simulink model "DC_MOTORControl2"  (R2021a)
settings: Solver=VariableStepAuto  StartTime=0.0  StopTime=1580  RelTol=1e-3
values from neighbouring files (symbols this model uses):
  B = 0.029    [MAIN.m]
  conv = 2*pi*2000    (= 12566.3706144)    [MAIN.m]
  J = 0.1    [MAIN.m]
  K = Ke    (= 0.6)    [MAIN.m]
  Ke = 0.6    [MAIN.m]
  Kt = 0.6    [MAIN.m]
  La = 1e-3    (= 0.001)    [MAIN.m]
  Ra = 1    [MAIN.m]
libraries: pid_lib x6, simulink x1
settings Model: Creator=Ferna  LastModifiedBy=Ferna

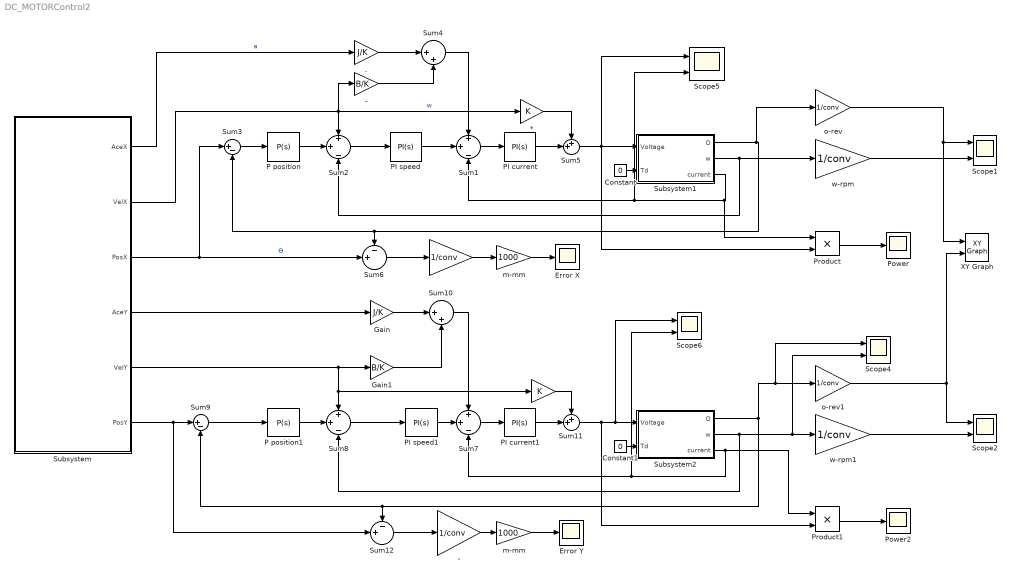
== system DC_MOTORControl2 ==
  " " : Gain  Gain=K
  "  " : Gain  Gain=1/conv
  ' : Gain  Gain=1/conv
  * : Gain  Gain=K
  - : Gain  Gain=B/K
  . : Gain  Gain=J/K
  Constant : Constant  Value=0
  Constant1 : Constant  Value=0
  Error X : Scope
  Error Y : Scope
  Gain : Gain  Gain=J/K
  Gain1 : Gain  Gain=B/K
  P position : pid_lib/PID Controller  Controller=P  Form=Parallel  TimeDomain=Continuous-time  UseExternalTs=off  SampleTime=-1  IntegratorMethod=Forward Euler  FilterMethod=Forward Euler  ControllerParametersSource=internal  P=1.1  I=B*5  D=0  UseFilter=on  N=100  TunerSelectOption=Transfer Function Based (PID Tuner App)  InitialConditionSource=internal  InitialConditionForIntegrator=0  InitialConditionForFilter=0  DifferentiatorICPrevScaledInput=0  ExternalReset=none  TrackingMode=off  Kt=1  LimitOutput=off  SatLimitsSource=internal  UpperSaturationLimit=inf  LowerSaturationLimit=-inf  LinearizeAsGain=on  AntiWindupMode=none  Kb=1  POutMin=[]  POutMax=[]  IOutMin=[]  IOutMax=[]  DOutMin=[]  DOutMax=[]  NOutMin=[]  NOutMax=[]  SumOutMin=[]  SumOutMax=[]  SaturationOutMin=[]  SaturationOutMax=[]  PParamMin=[]  PParamMax=[]  IParamMin=[]  IParamMax=[]  DParamMin=[]  DParamMax=[]  NParamMin=[]  NParamMax=[]  KbParamMin=[]  KbParamMax=[]  KtParamMin=[]  KtParamMax=[]  KbOutMin=[]  KbOutMax=[]  KtOutMin=[]  KtOutMax=[]  IntegratorOutMin=[]  IntegratorOutMax=[]  FilterOutMin=[]  FilterOutMax=[]  SumI1OutMin=[]  SumI1OutMax=[]  SumI2OutMin=[]  SumI2OutMax=[]  SumI3OutMin=[]  SumI3OutMax=[]  SumI4OutMin=[]  SumI4OutMax=[]  SumDOutMin=[]  SumDOutMax=[]  DifferentiatorOutMin=[]  DifferentiatorOutMax=[]  FilterDiffOutCoefMin=[]  FilterDiffOutCoefMax=[]  ReciprocalOutMin=[]  ReciprocalOutMax=[]  SumDenOutMin=[]  SumDenOutMax=[]  SumNumOutMin=[]  SumNumOutMax=[]  DivideOutMin=[]  DivideOutMax=[]  UdiffTsProdOutMin=[]  UdiffTsProdOutMax=[]  NTsProdOutMin=[]  NTsProdOutMax=[]  UintegralTsProdOutMin=[]  UintegralTsProdOutMax=[]  UngainTsProdOutMin=[]  UngainTsProdOutMax=[]  IntegratorContinuousStateAttributes=''  IntegratorStateMustResolveToSignalObject=off  IntegratorRTWStateStorageClass=Auto  FilterContinuousStateAttributes=''  FilterStateMustResolveToSignalObject=off  FilterRTWStateStorageClass=Auto  ParallelPVariant=InternalParameters  IdealPVariant=Disabled  IVariant=Disabled  DVariant=Disabled  IntegratorVariant=Disabled  SatVariant=Disabled  AWVariant=Disabled  PCopyVariant=Disabled  TRVariant=Disabled  FdbkBlocksVariant=Forward  IdealPFdbkVariant=Disabled  SatFdbkVariant=Disabled  DerivativeFilterVariant=Disabled  NVariant=Disabled  NCopyVariant=Disabled_SignalSpec  FilterICVariant=Disabled  IntegratorICVariant=Disabled  ExternalResetVariant=Disabled  TRSumVariant=Passthrough  SumFdbkVariant=Disabled  SumVariant=Passthrough_P  TsampFilterVariant=InternalTs  TsampNgainVariant=Passthrough  TsampIntegralVariant=Disabled_SignalSpec  ExternalSaturationOutDataTypeStr=Inherit: Same as second input
  P position1 : pid_lib/PID Controller  Controller=P  Form=Parallel  TimeDomain=Continuous-time  UseExternalTs=off  SampleTime=-1  IntegratorMethod=Forward Euler  FilterMethod=Forward Euler  ControllerParametersSource=internal  P=1.1  I=B*5  D=0  UseFilter=on  N=100  TunerSelectOption=Transfer Function Based (PID Tuner App)  InitialConditionSource=internal  InitialConditionForIntegrator=0  InitialConditionForFilter=0  DifferentiatorICPrevScaledInput=0  ExternalReset=none  TrackingMode=off  Kt=1  LimitOutput=off  SatLimitsSource=internal  UpperSaturationLimit=inf  LowerSaturationLimit=-inf  LinearizeAsGain=on  AntiWindupMode=none  Kb=1  POutMin=[]  POutMax=[]  IOutMin=[]  IOutMax=[]  DOutMin=[]  DOutMax=[]  NOutMin=[]  NOutMax=[]  SumOutMin=[]  SumOutMax=[]  SaturationOutMin=[]  SaturationOutMax=[]  PParamMin=[]  PParamMax=[]  IParamMin=[]  IParamMax=[]  DParamMin=[]  DParamMax=[]  NParamMin=[]  NParamMax=[]  KbParamMin=[]  KbParamMax=[]  KtParamMin=[]  KtParamMax=[]  KbOutMin=[]  KbOutMax=[]  KtOutMin=[]  KtOutMax=[]  IntegratorOutMin=[]  IntegratorOutMax=[]  FilterOutMin=[]  FilterOutMax=[]  SumI1OutMin=[]  SumI1OutMax=[]  SumI2OutMin=[]  SumI2OutMax=[]  SumI3OutMin=[]  SumI3OutMax=[]  SumI4OutMin=[]  SumI4OutMax=[]  SumDOutMin=[]  SumDOutMax=[]  DifferentiatorOutMin=[]  DifferentiatorOutMax=[]  FilterDiffOutCoefMin=[]  FilterDiffOutCoefMax=[]  ReciprocalOutMin=[]  ReciprocalOutMax=[]  SumDenOutMin=[]  SumDenOutMax=[]  SumNumOutMin=[]  SumNumOutMax=[]  DivideOutMin=[]  DivideOutMax=[]  UdiffTsProdOutMin=[]  UdiffTsProdOutMax=[]  NTsProdOutMin=[]  NTsProdOutMax=[]  UintegralTsProdOutMin=[]  UintegralTsProdOutMax=[]  UngainTsProdOutMin=[]  UngainTsProdOutMax=[]  IntegratorContinuousStateAttributes=''  IntegratorStateMustResolveToSignalObject=off  IntegratorRTWStateStorageClass=Auto  FilterContinuousStateAttributes=''  FilterStateMustResolveToSignalObject=off  FilterRTWStateStorageClass=Auto  ParallelPVariant=InternalParameters  IdealPVariant=Disabled  IVariant=Disabled  DVariant=Disabled  IntegratorVariant=Disabled  SatVariant=Disabled  AWVariant=Disabled  PCopyVariant=Disabled  TRVariant=Disabled  FdbkBlocksVariant=Forward  IdealPFdbkVariant=Disabled  SatFdbkVariant=Disabled  DerivativeFilterVariant=Disabled  NVariant=Disabled  NCopyVariant=Disabled_SignalSpec  FilterICVariant=Disabled  IntegratorICVariant=Disabled  ExternalResetVariant=Disabled  TRSumVariant=Passthrough  SumFdbkVariant=Disabled  SumVariant=Passthrough_P  TsampFilterVariant=InternalTs  TsampNgainVariant=Passthrough  TsampIntegralVariant=Disabled_SignalSpec  ExternalSaturationOutDataTypeStr=Inherit: Same as second input
  PI current : pid_lib/PID Controller  Controller=PI  Form=Parallel  TimeDomain=Continuous-time  UseExternalTs=off  SampleTime=-1  IntegratorMethod=Forward Euler  FilterMethod=Forward Euler  ControllerParametersSource=internal  P=La*1000  I=Ra*1000  D=0  UseFilter=on  N=100  TunerSelectOption=Transfer Function Based (PID Tuner App)  InitialConditionSource=internal  InitialConditionForIntegrator=0  InitialConditionForFilter=0  DifferentiatorICPrevScaledInput=0  ExternalReset=none  TrackingMode=off  Kt=1  LimitOutput=off  SatLimitsSource=internal  UpperSaturationLimit=inf  LowerSaturationLimit=-inf  LinearizeAsGain=on  AntiWindupMode=none  Kb=1  POutMin=[]  POutMax=[]  IOutMin=[]  IOutMax=[]  DOutMin=[]  DOutMax=[]  NOutMin=[]  NOutMax=[]  SumOutMin=[]  SumOutMax=[]  SaturationOutMin=[]  SaturationOutMax=[]  PParamMin=[]  PParamMax=[]  IParamMin=[]  IParamMax=[]  DParamMin=[]  DParamMax=[]  NParamMin=[]  NParamMax=[]  KbParamMin=[]  KbParamMax=[]  KtParamMin=[]  KtParamMax=[]  KbOutMin=[]  KbOutMax=[]  KtOutMin=[]  KtOutMax=[]  IntegratorOutMin=[]  IntegratorOutMax=[]  FilterOutMin=[]  FilterOutMax=[]  SumI1OutMin=[]  SumI1OutMax=[]  SumI2OutMin=[]  SumI2OutMax=[]  SumI3OutMin=[]  SumI3OutMax=[]  SumI4OutMin=[]  SumI4OutMax=[]  SumDOutMin=[]  SumDOutMax=[]  DifferentiatorOutMin=[]  DifferentiatorOutMax=[]  FilterDiffOutCoefMin=[]  FilterDiffOutCoefMax=[]  ReciprocalOutMin=[]  ReciprocalOutMax=[]  SumDenOutMin=[]  SumDenOutMax=[]  SumNumOutMin=[]  SumNumOutMax=[]  DivideOutMin=[]  DivideOutMax=[]  UdiffTsProdOutMin=[]  UdiffTsProdOutMax=[]  NTsProdOutMin=[]  NTsProdOutMax=[]  UintegralTsProdOutMin=[]  UintegralTsProdOutMax=[]  UngainTsProdOutMin=[]  UngainTsProdOutMax=[]  IntegratorContinuousStateAttributes=''  IntegratorStateMustResolveToSignalObject=off  IntegratorRTWStateStorageClass=Auto  FilterContinuousStateAttributes=''  FilterStateMustResolveToSignalObject=off  FilterRTWStateStorageClass=Auto  ParallelPVariant=InternalParameters  IdealPVariant=Disabled  IVariant=InternalParameters  DVariant=Disabled  IntegratorVariant=Continuous  SatVariant=Disabled  AWVariant=Passthrough  PCopyVariant=Disabled  TRVariant=Disabled  FdbkBlocksVariant=Forward  IdealPFdbkVariant=Disabled  SatFdbkVariant=Disabled  DerivativeFilterVariant=Disabled  NVariant=Disabled  NCopyVariant=Disabled_SignalSpec  FilterICVariant=Disabled  IntegratorICVariant=InternalICs  ExternalResetVariant=Disabled  TRSumVariant=Passthrough  SumFdbkVariant=Disabled  SumVariant=Sum_PI  TsampFilterVariant=InternalTs  TsampNgainVariant=Passthrough  TsampIntegralVariant=Passthrough  ExternalSaturationOutDataTypeStr=Inherit: Same as second input
  PI current1 : pid_lib/PID Controller  Controller=PI  Form=Parallel  TimeDomain=Continuous-time  UseExternalTs=off  SampleTime=-1  IntegratorMethod=Forward Euler  FilterMethod=Forward Euler  ControllerParametersSource=internal  P=La*1000  I=Ra*1000  D=0  UseFilter=on  N=100  TunerSelectOption=Transfer Function Based (PID Tuner App)  InitialConditionSource=internal  InitialConditionForIntegrator=0  InitialConditionForFilter=0  DifferentiatorICPrevScaledInput=0  ExternalReset=none  TrackingMode=off  Kt=1  LimitOutput=off  SatLimitsSource=internal  UpperSaturationLimit=inf  LowerSaturationLimit=-inf  LinearizeAsGain=on  AntiWindupMode=none  Kb=1  POutMin=[]  POutMax=[]  IOutMin=[]  IOutMax=[]  DOutMin=[]  DOutMax=[]  NOutMin=[]  NOutMax=[]  SumOutMin=[]  SumOutMax=[]  SaturationOutMin=[]  SaturationOutMax=[]  PParamMin=[]  PParamMax=[]  IParamMin=[]  IParamMax=[]  DParamMin=[]  DParamMax=[]  NParamMin=[]  NParamMax=[]  KbParamMin=[]  KbParamMax=[]  KtParamMin=[]  KtParamMax=[]  KbOutMin=[]  KbOutMax=[]  KtOutMin=[]  KtOutMax=[]  IntegratorOutMin=[]  IntegratorOutMax=[]  FilterOutMin=[]  FilterOutMax=[]  SumI1OutMin=[]  SumI1OutMax=[]  SumI2OutMin=[]  SumI2OutMax=[]  SumI3OutMin=[]  SumI3OutMax=[]  SumI4OutMin=[]  SumI4OutMax=[]  SumDOutMin=[]  SumDOutMax=[]  DifferentiatorOutMin=[]  DifferentiatorOutMax=[]  FilterDiffOutCoefMin=[]  FilterDiffOutCoefMax=[]  ReciprocalOutMin=[]  ReciprocalOutMax=[]  SumDenOutMin=[]  SumDenOutMax=[]  SumNumOutMin=[]  SumNumOutMax=[]  DivideOutMin=[]  DivideOutMax=[]  UdiffTsProdOutMin=[]  UdiffTsProdOutMax=[]  NTsProdOutMin=[]  NTsProdOutMax=[]  UintegralTsProdOutMin=[]  UintegralTsProdOutMax=[]  UngainTsProdOutMin=[]  UngainTsProdOutMax=[]  IntegratorContinuousStateAttributes=''  IntegratorStateMustResolveToSignalObject=off  IntegratorRTWStateStorageClass=Auto  FilterContinuousStateAttributes=''  FilterStateMustResolveToSignalObject=off  FilterRTWStateStorageClass=Auto  ParallelPVariant=InternalParameters  IdealPVariant=Disabled  IVariant=InternalParameters  DVariant=Disabled  IntegratorVariant=Continuous  SatVariant=Disabled  AWVariant=Passthrough  PCopyVariant=Disabled  TRVariant=Disabled  FdbkBlocksVariant=Forward  IdealPFdbkVariant=Disabled  SatFdbkVariant=Disabled  DerivativeFilterVariant=Disabled  NVariant=Disabled  NCopyVariant=Disabled_SignalSpec  FilterICVariant=Disabled  IntegratorICVariant=InternalICs  ExternalResetVariant=Disabled  TRSumVariant=Passthrough  SumFdbkVariant=Disabled  SumVariant=Sum_PI  TsampFilterVariant=InternalTs  TsampNgainVariant=Passthrough  TsampIntegralVariant=Passthrough  ExternalSaturationOutDataTypeStr=Inherit: Same as second input
  PI speed : pid_lib/PID Controller  Controller=PI  Form=Parallel  TimeDomain=Continuous-time  UseExternalTs=off  SampleTime=-1  IntegratorMethod=Forward Euler  FilterMethod=Forward Euler  ControllerParametersSource=internal  P=J*10  I=B*10  D=0  UseFilter=on  N=100  TunerSelectOption=Transfer Function Based (PID Tuner App)  InitialConditionSource=internal  InitialConditionForIntegrator=0  InitialConditionForFilter=0  DifferentiatorICPrevScaledInput=0  ExternalReset=none  TrackingMode=off  Kt=1  LimitOutput=off  SatLimitsSource=internal  UpperSaturationLimit=inf  LowerSaturationLimit=-inf  LinearizeAsGain=on  AntiWindupMode=none  Kb=1  POutMin=[]  POutMax=[]  IOutMin=[]  IOutMax=[]  DOutMin=[]  DOutMax=[]  NOutMin=[]  NOutMax=[]  SumOutMin=[]  SumOutMax=[]  SaturationOutMin=[]  SaturationOutMax=[]  PParamMin=[]  PParamMax=[]  IParamMin=[]  IParamMax=[]  DParamMin=[]  DParamMax=[]  NParamMin=[]  NParamMax=[]  KbParamMin=[]  KbParamMax=[]  KtParamMin=[]  KtParamMax=[]  KbOutMin=[]  KbOutMax=[]  KtOutMin=[]  KtOutMax=[]  IntegratorOutMin=[]  IntegratorOutMax=[]  FilterOutMin=[]  FilterOutMax=[]  SumI1OutMin=[]  SumI1OutMax=[]  SumI2OutMin=[]  SumI2OutMax=[]  SumI3OutMin=[]  SumI3OutMax=[]  SumI4OutMin=[]  SumI4OutMax=[]  SumDOutMin=[]  SumDOutMax=[]  DifferentiatorOutMin=[]  DifferentiatorOutMax=[]  FilterDiffOutCoefMin=[]  FilterDiffOutCoefMax=[]  ReciprocalOutMin=[]  ReciprocalOutMax=[]  SumDenOutMin=[]  SumDenOutMax=[]  SumNumOutMin=[]  SumNumOutMax=[]  DivideOutMin=[]  DivideOutMax=[]  UdiffTsProdOutMin=[]  UdiffTsProdOutMax=[]  NTsProdOutMin=[]  NTsProdOutMax=[]  UintegralTsProdOutMin=[]  UintegralTsProdOutMax=[]  UngainTsProdOutMin=[]  UngainTsProdOutMax=[]  IntegratorContinuousStateAttributes=''  IntegratorStateMustResolveToSignalObject=off  IntegratorRTWStateStorageClass=Auto  FilterContinuousStateAttributes=''  FilterStateMustResolveToSignalObject=off  FilterRTWStateStorageClass=Auto  ParallelPVariant=InternalParameters  IdealPVariant=Disabled  IVariant=InternalParameters  DVariant=Disabled  IntegratorVariant=Continuous  SatVariant=Disabled  AWVariant=Passthrough  PCopyVariant=Disabled  TRVariant=Disabled  FdbkBlocksVariant=Forward  IdealPFdbkVariant=Disabled  SatFdbkVariant=Disabled  DerivativeFilterVariant=Disabled  NVariant=Disabled  NCopyVariant=Disabled_SignalSpec  FilterICVariant=Disabled  IntegratorICVariant=InternalICs  ExternalResetVariant=Disabled  TRSumVariant=Passthrough  SumFdbkVariant=Disabled  SumVariant=Sum_PI  TsampFilterVariant=InternalTs  TsampNgainVariant=Passthrough  TsampIntegralVariant=Passthrough  ExternalSaturationOutDataTypeStr=Inherit: Same as second input
  PI speed1 : pid_lib/PID Controller  Controller=PI  Form=Parallel  TimeDomain=Continuous-time  UseExternalTs=off  SampleTime=-1  IntegratorMethod=Forward Euler  FilterMethod=Forward Euler  ControllerParametersSource=internal  P=J*10  I=B*10  D=0  UseFilter=on  N=100  TunerSelectOption=Transfer Function Based (PID Tuner App)  InitialConditionSource=internal  InitialConditionForIntegrator=0  InitialConditionForFilter=0  DifferentiatorICPrevScaledInput=0  ExternalReset=none  TrackingMode=off  Kt=1  LimitOutput=off  SatLimitsSource=internal  UpperSaturationLimit=inf  LowerSaturationLimit=-inf  LinearizeAsGain=on  AntiWindupMode=none  Kb=1  POutMin=[]  POutMax=[]  IOutMin=[]  IOutMax=[]  DOutMin=[]  DOutMax=[]  NOutMin=[]  NOutMax=[]  SumOutMin=[]  SumOutMax=[]  SaturationOutMin=[]  SaturationOutMax=[]  PParamMin=[]  PParamMax=[]  IParamMin=[]  IParamMax=[]  DParamMin=[]  DParamMax=[]  NParamMin=[]  NParamMax=[]  KbParamMin=[]  KbParamMax=[]  KtParamMin=[]  KtParamMax=[]  KbOutMin=[]  KbOutMax=[]  KtOutMin=[]  KtOutMax=[]  IntegratorOutMin=[]  IntegratorOutMax=[]  FilterOutMin=[]  FilterOutMax=[]  SumI1OutMin=[]  SumI1OutMax=[]  SumI2OutMin=[]  SumI2OutMax=[]  SumI3OutMin=[]  SumI3OutMax=[]  SumI4OutMin=[]  SumI4OutMax=[]  SumDOutMin=[]  SumDOutMax=[]  DifferentiatorOutMin=[]  DifferentiatorOutMax=[]  FilterDiffOutCoefMin=[]  FilterDiffOutCoefMax=[]  ReciprocalOutMin=[]  ReciprocalOutMax=[]  SumDenOutMin=[]  SumDenOutMax=[]  SumNumOutMin=[]  SumNumOutMax=[]  DivideOutMin=[]  DivideOutMax=[]  UdiffTsProdOutMin=[]  UdiffTsProdOutMax=[]  NTsProdOutMin=[]  NTsProdOutMax=[]  UintegralTsProdOutMin=[]  UintegralTsProdOutMax=[]  UngainTsProdOutMin=[]  UngainTsProdOutMax=[]  IntegratorContinuousStateAttributes=''  IntegratorStateMustResolveToSignalObject=off  IntegratorRTWStateStorageClass=Auto  FilterContinuousStateAttributes=''  FilterStateMustResolveToSignalObject=off  FilterRTWStateStorageClass=Auto  ParallelPVariant=InternalParameters  IdealPVariant=Disabled  IVariant=InternalParameters  DVariant=Disabled  IntegratorVariant=Continuous  SatVariant=Disabled  AWVariant=Passthrough  PCopyVariant=Disabled  TRVariant=Disabled  FdbkBlocksVariant=Forward  IdealPFdbkVariant=Disabled  SatFdbkVariant=Disabled  DerivativeFilterVariant=Disabled  NVariant=Disabled  NCopyVariant=Disabled_SignalSpec  FilterICVariant=Disabled  IntegratorICVariant=InternalICs  ExternalResetVariant=Disabled  TRSumVariant=Passthrough  SumFdbkVariant=Disabled  SumVariant=Sum_PI  TsampFilterVariant=InternalTs  TsampNgainVariant=Passthrough  TsampIntegralVariant=Passthrough  ExternalSaturationOutDataTypeStr=Inherit: Same as second input
  Power : Scope
  Power2 : Scope
  Product : Product
  Product1 : Product
  Scope{1..2,4..6} (5 alike) : Scope  NumInputPorts=2
  Subsystem : Subsystem
  Subsystem1 : Subsystem
  Subsystem2 : Subsystem
  Sum{1..2,7..8} (4 alike) : Sum  Inputs=+|+|-
  Sum10 : Sum  Inputs=|++
  Sum11 : Sum  Inputs=++|
  Sum12 : Sum  Inputs=-+|
  Sum3 : Sum  Inputs=|+-
  Sum4 : Sum  Inputs=|++
  Sum5 : Sum  Inputs=++|
  Sum6 : Sum  Inputs=-+|
  Sum9 : Sum  Inputs=|+-
  XY Graph : simulink/Sinks/XY Graph  xmin=0  xmax=3  ymin=0  ymax=2  st=1
  m-mm : Gain  Gain=1000
  "m-mm " : Gain  Gain=1000
  o-rev : Gain  Gain=1/conv
  o-rev1 : Gain  Gain=1/conv
  w-rpm : Gain  Gain=1/conv
  w-rpm1 : Gain  Gain=1/conv
  wires:
  o-rev/1 -> XY Graph/1, Scope1/1
  Subsystem1/2(w) -> w-rpm/1, Sum2/3
  w-rpm/1 -> Scope1/2
  Constant/1 -> Subsystem1/2(Td)
  Sum1/1 -> PI current/1
  Sum2/1 -> PI speed/1
  Sum3/1 -> P position/1
  Subsystem1/3(current) -> Product/1, Scope5/2, Sum1/3
  PI speed/1 -> Sum1/2
  Subsystem/3(PosX) -> Sum3/1, Sum6/2  "ϴ"
  PI current/1 -> Sum5/2
  Sum5/1 -> Scope5/1, Product/2, Subsystem1/1(Voltage)
  P position/1 -> Sum2/2
  Product/1 -> Power/1
  Sum12/1 -> '/1
  Product1/1 -> Power2/1
  Subsystem2/2(w) -> Sum8/3, Scope4/2, w-rpm1/1
  Subsystem2/1(O) -> Scope4/1, o-rev1/1, Sum12/1, Sum9/2
  Gain/1 -> Sum10/1
  Subsystem/5(VelY) -> Gain1/1, Sum8/1, " "/1
  " "/1 -> Sum11/1
  Subsystem2/3(current) -> Scope6/2, Sum7/3, Product1/1
  Sum7/1 -> PI current1/1
  PI speed1/1 -> Sum7/2
  Gain1/1 -> Sum10/2
  PI current1/1 -> Sum11/2
  Constant1/1 -> Subsystem2/2(Td)
  Sum8/1 -> PI speed1/1
  o-rev1/1 -> Scope2/1, XY Graph/2
  Sum10/1 -> Sum7/1
  Sum9/1 -> P position1/1
  Sum11/1 -> Scope6/1, Subsystem2/1(Voltage), Product1/2
  P position1/1 -> Sum8/2
  ./1 -> Sum4/1
  Subsystem/2(VelX) -> Sum2/1, */1, -/1  "w"
  -/1 -> Sum4/2
  */1 -> Sum5/1
  Sum4/1 -> Sum1/1
  Subsystem/1(AceX) -> ./1  "a"
  Subsystem1/1(O) -> o-rev/1, Sum6/1, Sum3/2
  Sum6/1 -> "  "/1
  Subsystem/6(PosY) -> Sum12/2, Sum9/1
  Subsystem/4(AceY) -> Gain/1
  w-rpm1/1 -> Scope2/2
  "  "/1 -> m-mm/1
  m-mm/1 -> Error X/1
  '/1 -> "m-mm "/1
  "m-mm "/1 -> Error Y/1

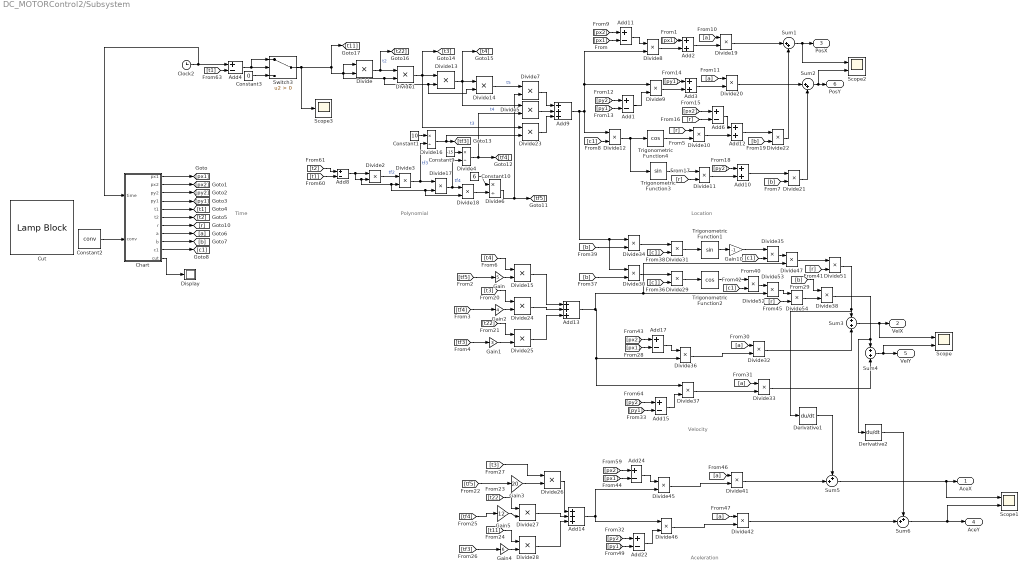
== system DC_MOTORControl2/Subsystem ==
  note: Polynomial
  note: Location
  note: Time
  note: Velocity
  note: Aceleration
  Add{1,4,6,8,11,15,17,22,24} (9 alike) : Sum  Inputs=+-
  Add{2..3,10,12} (4 alike) : Sum
  Add13 : Sum  Inputs=+++
  Add14 : Sum  Inputs=+++
  Add9 : Sum  Inputs=+++
  Chart : Stateflow chart  TreatAsAtomicUnit=on
  Clock2 : Clock
  Constant1 : Constant  Value=10
  Constant10 : Constant  Value=6
  Constant2 : Constant  Value=conv
  Constant3 : Constant  Value=0
  Constant9 : Constant  Value=-15
  Cut : LampBlock
  Derivative1 : Derivative
  Derivative2 : Derivative
  Display : Display
  Divide{,1..3,5,7..15,17..38,41..42,45..47,51..54} (45 alike) : Product  Inputs=**
  Divide16 : Product  Inputs=*/
  Divide4 : Product  Inputs=*/
  Divide6 : Product  Inputs=*/
  Gain : Gain  Gain=5
  Gain1 : Gain  Gain=3
  Gain10 : Gain  Gain=-1
  Gain2 : Gain  Gain=4
  Gain3 : Gain  Gain=20
  Gain4 : Gain  Gain=6
  Gain5 : Gain  Gain=12
  Scope : Scope  NumInputPorts=2
  Scope1 : Scope  NumInputPorts=2
  Scope2 : Scope  NumInputPorts=2
  Scope3 : Scope
  Sum1 : Sum  Inputs=|++
  Sum2 : Sum  Inputs=|++
  Sum3 : Sum  Inputs=+|+
  Sum4 : Sum  Inputs=+|+
  Sum5 : Sum  Inputs=++|
  Sum6 : Sum  Inputs=++|
  Switch3 : Switch  Criteria=u2 > Threshold
  Trigonometric Function1 : Trigonometry
  Trigonometric Function2 : Trigonometry  Operator=cos
  Trigonometric Function3 : Trigonometry
  Trigonometric Function4 : Trigonometry  Operator=cos
  AceX : Outport
  VelX : Outport  Port=2
  PosX : Outport  Port=3
  AceY : Outport  Port=4
  VelY : Outport  Port=5
  PosY : Outport  Port=6
  wires:
  Add3/1 -> Divide20/2
  Clock2/1 -> Chart/1(time), Add4/1
  Add8/1 -> Divide18/2, Divide17/2, Divide3/2, Divide2/2, Divide2/1
  Switch3/1 -> Divide14/2, Divide13/2, Divide1/2, Divide/2, Divide/1, [t11], Scope3/1
  [a] -> Divide19/1
  [t2] -> Add8/1
  Constant10/1 -> Divide6/1
  Add10/1 -> Divide21/1
  [c1] -> Divide12/2
  Constant9/1 -> Divide4/1
  [px1] -> Add2/1
  [t1] -> Add4/2
  [b] -> Divide22/2
  Divide7/1 -> Add9/1
  Divide12/1 -> Trigonometric Function3/1, Trigonometric Function4/1
  Divide18/1 -> Divide6/2
  Add4/1 -> Switch3/1, Switch3/2
  Divide2/1 -> Divide3/1  "tf2"
  Divide9/1 -> Add3/2
  Trigonometric Function3/1 -> Divide11/1
  Add2/1 -> Divide19/2
  Divide13/1 -> [t4], Divide14/1, Divide5/1  "t4"
  Divide20/1 -> Sum2/1
  [a] -> Divide20/1
  Divide19/1 -> Sum1/1
  Trigonometric Function4/1 -> Divide10/2
  Divide23/1 -> Add9/3
  Divide5/1 -> Add9/2
  [px2] -> Add6/1
  Add1/1 -> Divide9/2
  Divide8/1 -> Add2/2
  [b] -> Divide21/2
  Divide1/1 -> [t3], Divide13/1, Divide23/1  "t3"
  Constant3/1 -> Switch3/3
  Divide14/1 -> Divide7/1  "t5"
  Divide3/1 -> Divide16/2, Divide17/1  "tf3"
  Add12/1 -> Divide22/1
  Constant1/1 -> Divide16/1
  Divide/1 -> [t22], Divide1/1  "t2"
  Divide17/1 -> Divide4/2, Divide18/1  "tf4"
  [r] -> Divide11/2
  Divide6/1 -> [tf5], Divide7/2
  Divide4/1 -> [tf4], Divide5/2
  Divide16/1 -> [tf3], Divide23/2
  Chart/1(px1) -> [px1]
  Chart/2(px2) -> [px2]
  Chart/3(py2) -> [py2]
  Chart/4(py1) -> [py1]
  Chart/5(t1) -> [t1]
  Chart/6(t2) -> [t2]
  Chart/7(r) -> [r]
  Chart/8(a) -> [a]
  Chart/9(b) -> [b]
  Chart/10(c1) -> [c1]
  Chart/11(cut) -> Display/1
  [px1] -> Add11/2
  [px2] -> Add11/1
  Add11/1 -> Divide8/1
  [py1] -> Add1/2
  [py1] -> Add3/1
  [r] -> Add6/2
  [r] -> Divide10/1
  [py2] -> Add10/1
  Add6/1 -> Add12/1
  [tf5] -> Gain/1
  Gain/1 -> Divide15/2
  [t4] -> Divide15/1
  [tf4] -> Gain2/1
  [t3] -> Divide24/1
  Gain2/1 -> Divide24/2
  [t22] -> Divide25/1
  Gain1/1 -> Divide25/2
  [tf3] -> Gain1/1
  Divide15/1 -> Add13/1
  Divide24/1 -> Add13/2
  Divide25/1 -> Add13/3
  [tf5] -> Gain3/1
  [tf3] -> Gain4/1
  Gain5/1 -> Divide27/2
  [t22] -> Divide27/1
  [tf4] -> Gain5/1
  Divide27/1 -> Add14/2
  Divide26/1 -> Add14/1
  Gain3/1 -> Divide26/2
  [t11] -> Divide28/1
  Divide28/1 -> Add14/3
  Gain4/1 -> Divide28/2
  [t3] -> Divide26/1
  [py1] -> Add15/2
  [px2] -> Add17/1
  [px1] -> Add17/2
  [py2] -> Add15/1
  Add17/1 -> Divide36/1
  [a] -> Divide32/1
  [a] -> Divide33/1
  Add15/1 -> Divide37/2
  [py1] -> Add22/2
  [px2] -> Add24/1
  [px1] -> Add24/2
  Add14/1 -> Divide46/1, Divide45/2
  [py2] -> Add22/1
  Add24/1 -> Divide45/1
  Divide45/1 -> Divide41/2
  [a] -> Divide41/1
  [a] -> Divide42/1
  Add22/1 -> Divide46/2
  Divide46/1 -> Divide42/2
  [t1] -> Add8/2
  [py2] -> Add1/1
  Divide36/1 -> Divide32/2
  Divide37/1 -> Divide33/2
  Constant2/1 -> Chart/2(conv)
  Divide22/1 -> Sum1/2
  Divide21/1 -> Sum2/2
  Divide11/1 -> Add10/2
  Divide32/1 -> Sum3/2
  Divide33/1 -> Sum4/2
  Trigonometric Function1/1 -> Gain10/1
  Divide34/1 -> Divide31/1
  [c1] -> Divide31/2
  Divide31/1 -> Trigonometric Function1/1
  Add9/1 -> Divide9/1, Divide8/2, Divide12/1, Divide30/1, Divide34/1
  [b] -> Divide34/2
  Gain10/1 -> Divide35/1
  [c1] -> Divide35/2
  Divide47/1 -> Divide51/1
  [r] -> Divide51/2
  Divide35/1 -> Divide47/1
  [c1] -> Divide52/2
  Divide29/1 -> Trigonometric Function2/1
  Add13/1 -> Divide37/1, Divide36/2, Divide47/2, Divide53/2
  [r] -> Divide54/2
  Divide30/1 -> Divide29/1
  Divide52/1 -> Divide53/1
  [c1] -> Divide29/2
  Divide53/1 -> Divide54/1
  [b] -> Divide30/2
  Trigonometric Function2/1 -> Divide52/1
  Divide51/1 -> Derivative1/1, Sum3/1
  Divide41/1 -> Sum5/2
  Derivative1/1 -> Sum5/1
  Divide42/1 -> Sum6/2
  Derivative2/1 -> Sum6/1
  [b] -> Divide38/1
  Divide54/1 -> Divide38/2
  Divide38/1 -> Derivative2/1, Sum4/1
  Divide10/1 -> Add12/2
  Sum1/1 -> Scope2/1, PosX/1
  Sum2/1 -> Scope2/2, PosY/1
  Sum3/1 -> Scope/1, VelX/1
  Sum4/1 -> Scope/2, VelY/1
  Sum5/1 -> Scope1/1, AceX/1
  Sum6/1 -> Scope1/2, AceY/1

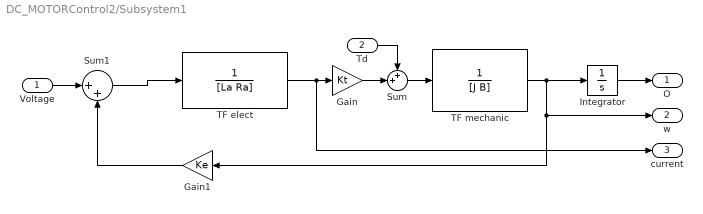
== system DC_MOTORControl2/Subsystem1 ==
  Voltage : Inport
  Td : Inport  Port=2
  Gain : Gain  Gain=Kt
  Gain1 : Gain  Gain=Ke
  Integrator : Integrator
  Sum : Sum  Inputs=++|
  Sum1 : Sum  Inputs=|++
  TF elect : TransferFcn  Denominator=[La Ra]
  TF mechanic : TransferFcn  Denominator=[J B]
  O : Outport
  w : Outport  Port=2
  current : Outport  Port=3
  wires:
  Integrator/1 -> O/1
  Sum1/1 -> TF elect/1
  Gain1/1 -> Sum1/2
  TF elect/1 -> current/1, Gain/1
  TF mechanic/1 -> w/1, Gain1/1, Integrator/1
  Voltage/1 -> Sum1/1
  Sum/1 -> TF mechanic/1
  Gain/1 -> Sum/2
  Td/1 -> Sum/1

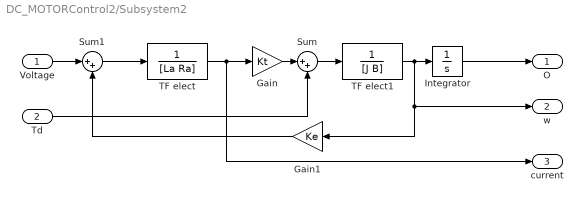
== system DC_MOTORControl2/Subsystem2 ==
  Voltage : Inport
  Td : Inport  Port=2
  Gain : Gain  Gain=Kt
  Gain1 : Gain  Gain=Ke
  Integrator : Integrator
  Sum : Sum  Inputs=|++
  Sum1 : Sum  Inputs=|++
  TF elect : TransferFcn  Denominator=[La Ra]
  TF elect1 : TransferFcn  Denominator=[J B]
  O : Outport
  w : Outport  Port=2
  current : Outport  Port=3
  wires:
  Integrator/1 -> O/1
  Sum1/1 -> TF elect/1
  Gain1/1 -> Sum1/2
  TF elect/1 -> current/1, Gain/1
  TF elect1/1 -> w/1, Gain1/1, Integrator/1
  Voltage/1 -> Sum1/1
  Gain/1 -> Sum/1
  Sum/1 -> TF elect1/1
  Td/1 -> Sum/2

== stateflow chart DC_MOTORControl2/Subsystem/Chart ==
  state posrest
    entry:
    px1=0;
    px2=3*conv;
    py1=0;
    py2=2*conv;
    t1=0;
    t2=270;
    a=1;
    b=0;
    cut=0;
  state post11
    entry:
    px1=2*conv;
    px2=3*conv;
    py1=1.4*conv;
    py2=2*conv;
    t1=1480;
    t2=1580;
    a=1;
    b=0
    cut=0;
  state post1
    entry:
    px1=3*conv;
    px2=0.2*conv;
    py1=2*conv;
    py2=0.4*conv;
    t1=270;
    t2=520;
    a=1;
    b=0;
    cut=0;
  state CIRCLE [group]
    state post10
      entry:
      r=0.4*conv;
      c1=2*pi;
      a=0;
      b=1;
      t1=1260;
      t2=1480;
      cut=1;
  state TRIANGLE [group]
    state post2
      entry:
      px1=0.2*conv;
      px2=1*conv;
      py1=0.4*conv;
      py2=0.4*conv;
      t1=520;
      t2=590;
      a=1;
      b=0;
      cut=1;
    state post5
      entry:
      px1=0.6*conv;
      px2=0.2*conv;
      py1=1.2*conv;
      py2=0.4*conv;
      t1=660;
      t2=730;
      a=1;
      b=0;
      cut=1;
    state post3
      entry:
      px1=1*conv;
      px2=0.6*conv;
      py1=0.4*conv;
      py2=1.2*conv;
      t1=590;
      t2=660;
      a=1;
      b=0;
      cut=1;
    post3 -> post5 : [time>660 && time<730]
    post2 -> post3 : [time>590 && time<660]
  state post9
    entry:
    px1=1.6*conv;
    px2=2*conv;
    py1=0.2*conv;
    py2=1.4*conv;
    t1=1155;
    t2=1260;
    a=1;
    b=0;
    cut=0;
  state SEMI_CIRCLE [group]
    state post8
      entry:
      t1=960;
      t2=1155;
      r=0.6*conv;
      c1=1*pi;
      a=0;
      b=1;
      cut=1;
    state post7
      entry:
      px1=1.6*conv;
      px2=2.8*conv;
      py1=0.2*conv;
      py2=0.2*conv;
      t1=855;
      t2=960;
      a=1;
      b=0;
      cut=1;
    post7 -> post8 : [time>960 && time<1155]
  state post6
    entry:
    px1=0.2*conv;
    px2=1.6*conv;
    py1=0.4*conv;
    py2=0.2*conv;
    t1=730;
    t2=855;
    a=1;
    b=0;
    cut=0;
  (default) -> posrest
  posrest -> post1 : [time>270 && time<520]
  post10 -> post11 : [time>1480 && time<1580]
  post1 -> post2 : [time>520 && time<590]
  post9 -> post10 : [time>1260 && time<1480]
  post5 -> post6 : [time>730 && time<855]
  post8 -> post9 : [time>1155 && time<1260]
  post6 -> post7 : [time>855 && time<960]
  data: px1 output; px2 output; py2 output; py1 output; t1 output; t2 output; r output; a output; b output; c1 output; time input; cut output; conv input
